simulink model "BuckBosstConverter"  (R2020a)
settings: Solver=FixedStepDiscrete  StartTime=0.0  StopTime=T  FixedStep=Ts  RelTol=1e-3
PreLoadFcn:
  | % Load all configuration
  | config;
values from neighbouring files (symbols this model uses):
  C = 3330e-6    (= 0.00333)    [config.m]
  C_PV = 0.05    [GridConnectedDesignConfiguration.m]    (also in config.m = 0.0001)
  L = 5e-3    (= 0.005)    [config.m]
  LOAD = 7    [config.m]
  R_PV = 10e-3    (= 0.01)    [GridConnectedDesignConfiguration.m]    (also in config.m)
  Rs = 0.1    [config.m]
  temp = 25    [config.m]
  Ts = 5e-6    (= 5e-06)    [GridConnectedDesignConfiguration.m]    (also in config.m = 1e-05)
undefined symbols (not defined in the file or in its folder): Ion, Lithium
libraries: powerlib x13, simulink x2, powerlib_meascontrol x2, electricdrivelib x1, re_lib x1, SignalEditorBlockLib x1
settings Model: Creator=debma  LastModifiedBy=debma

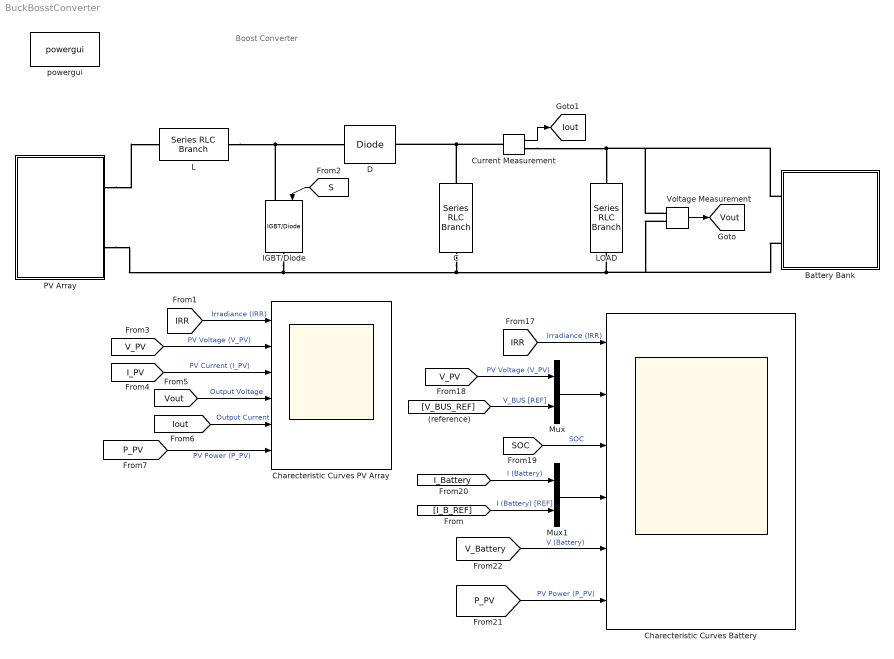
== system BuckBosstConverter ==
  note: Boost Converter
  Battery Bank : Subsystem
  C : powerlib/Elements/Series RLC Branch  LConnTagsString=__new0  RConnTagsString=__new0  BranchType=RC  Resistance=Rs  Inductance=L  SetiL0=off  InitialCurrent=0  Capacitance=C  Setx0=off  InitialVoltage=0  Measurements=None
  Charecteristic Curves Battery : Scope  NumInputPorts=6
  Charecteristic Curves PV Array : Scope  NumInputPorts=6
  Current Measurement : powerlib/Measurements/Current Measurement  PhasorSimulation=off  OutputType=Complex  PSBequivalent=0
  D : powerlib/Power Electronics/Diode  Ron=0.001  Lon=0  Vf=0.8  IC=0  UseSnubber=0  Rs=500  Cs=250e-9  Measurements=off
  IGBT/Diode : powerlib/Power Electronics/IGBT//Diode  Ron=1e-3  Rs=1e5  Cs=inf  Measurements=off
  L : powerlib/Elements/Series RLC Branch  LConnTagsString=__new0  RConnTagsString=__new0  BranchType=RL  Resistance=Rs  Inductance=L  SetiL0=off  InitialCurrent=0  Capacitance=1e-6  Setx0=off  InitialVoltage=0  Measurements=None
  LOAD : powerlib/Elements/Series RLC Branch  LConnTagsString=__new0  RConnTagsString=__new0  BranchType=R  Resistance=LOAD  Inductance=L  SetiL0=off  InitialCurrent=0  Capacitance=1e-6  Setx0=off  InitialVoltage=0  Measurements=None
  Mux : Mux  Inputs=2
  Mux1 : Mux  Inputs=2
  PV Array : Subsystem
  Voltage Measurement : powerlib/Measurements/Voltage Measurement  PhasorSimulation=off  OutputType=Complex  PSBequivalent=0
  powergui : powerlib/powergui  Priority=1  SimulationMode=Discrete  SampleTime=Ts  frequency=60  Iterations=50  frequencyindice=0  Pbase=100e6  ErrMax=1e-4  UnitsV=kV  UnitsW=MW  buscounter=0  FunctionMessages=off  echomessages=off  EnableUseOfTLC=off  CurrentSourceSwitches=off  DisableSnubberDevices=off  DisableRonSwitches=off  DisableVfSwitches=off  DisplayEquations=off  AutomaticDiscreteSolvers=off  SolverType=Tustin/Backward Euler (TBE)  Interpol=off  ExternalGateDelay=off  methode=off  Ts=100  x0status=blocks  SPID=on  SwTol=0  HookPort=off  NonlinearTolerance=1e-4  nMaxIteration=100  ContinueOnMaxIteration=off  RestoreLinks=warning  ResistiveCurrentMeasurement=off  Frange=[0:2:500]  Ylog=off  Xlog=on  ShowGrid=off  save=off  variable=ZData  structure=0  ZoomFFT=off  StartTime=0.0  cycles=1  DisplayStyle=1  fundamental=60  FreqAxis=off  MaxFrequency=1000  frequencyindicesteady=1  RmsSteady=1  display=off
  tag scope: Iout=global, Vout=global
  wires:
  Voltage Measurement/1 -> [Vout]
  Current Measurement/1 -> [Iout]
  [S] -> IGBT/Diode/1
  [V_PV] -> Charecteristic Curves PV Array/2  "PV Voltage (V_PV)"
  [IRR] -> Charecteristic Curves PV Array/1  "Irradiance (IRR)"
  [Vout] -> Charecteristic Curves PV Array/4  "Output Voltage"
  [Iout] -> Charecteristic Curves PV Array/5  "Output Current"
  [I_PV] -> Charecteristic Curves PV Array/3  "PV Current (I_PV)"
  [P_PV] -> Charecteristic Curves PV Array/6  "PV Power (P_PV)"
  Mux/1 -> Charecteristic Curves Battery/2
  [IRR] -> Charecteristic Curves Battery/1  "Irradiance (IRR)"
  [V_BUS_REF] -> Mux/2  "V_BUS [REF]"
  [I_B_REF] -> Mux1/2  "I (Battery) [REF]"
  [SOC] -> Charecteristic Curves Battery/3  "SOC"
  [I_Battery] -> Mux1/1  "I (Battery)"
  [V_Battery] -> Charecteristic Curves Battery/5  "V (Battery)"
  [V_PV] -> Mux/1  "PV Voltage (V_PV)"
  [P_PV] -> Charecteristic Curves Battery/6  "PV Power (P_PV)"
  Mux1/1 -> Charecteristic Curves Battery/4
  connections:
  PV Array/RConn1 -- L/LConn1
  PV Array/RConn2 -- IGBT/Diode/RConn1 -- Voltage Measurement/LConn2 -- Battery Bank/LConn2 -- LOAD/RConn1 -- C/RConn1
  L/RConn1 -- IGBT/Diode/LConn1 -- D/LConn1
  C/LConn1 -- D/RConn1 -- Current Measurement/LConn1
  Current Measurement/RConn1 -- Voltage Measurement/LConn1 -- Battery Bank/LConn1 -- LOAD/LConn1

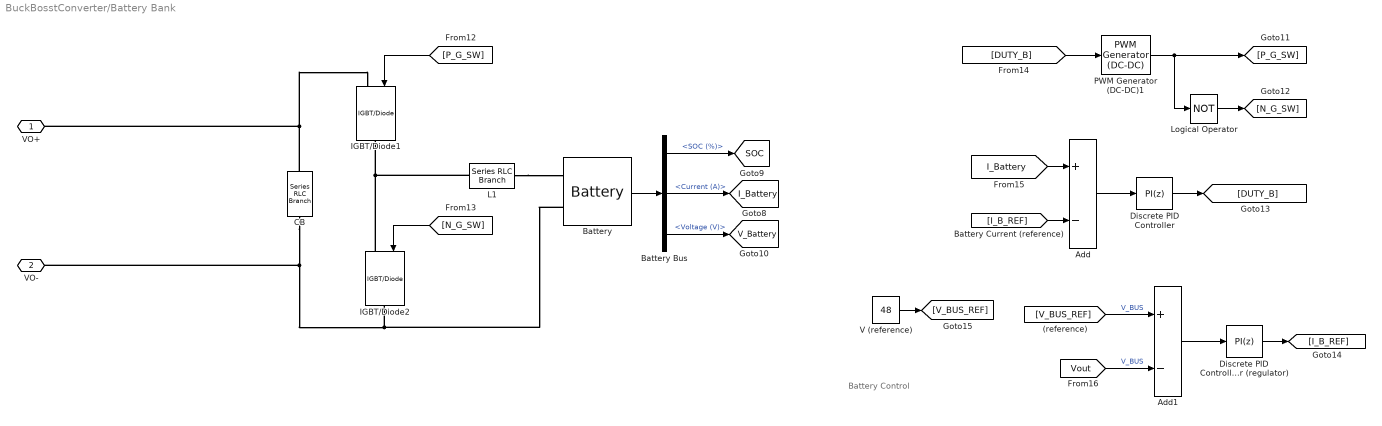
== system BuckBosstConverter/Battery Bank ==
  note: Battery Control
  Add : Sum  Inputs=+-
  Add1 : Sum  Inputs=+-
  Battery : electricdrivelib/Extra Sources/Battery  BatType=Lithium-Ion  ShowTempParam=off  ThermalPreset=no  ShowAgeParam=off  NomV=24  NomQ=50  SOC=45  Batt_Tr=1  PresetModel=on  MaxQ=50  MinV=18  FullV=27.9357  Dis_rate=21.7391  R=0.0048  Normal_OP=45.2174  expZone="[25.9293      2.45652]"  current=[6.5 13 32.5]  Units=Time  Tci=20  NomT=20  T2=-30  MaxQ2=4.8  FullV2=7.1  Normal_OP2=5.655  expZone2="[6.58           1]"  Rca=0.6  ti=2000  Dp=0  Neq0=0  Tsim=1e6  Ta1=25  Qeol=5.4*0.9  Reol=0.013333*1.2  Char_age=[2.3478, 3]  Dis_age=[2.3478, 10]  N1=1500  N2=10500  N3=1000  N4=1400  Ta2=45  N5=950
  Battery Bus : BusSelector  OutputSignals=SOC (%),Current (A),Voltage (V)
  CB : powerlib/Elements/Series RLC Branch  LConnTagsString=__new0  RConnTagsString=__new0  BranchType=RC  Resistance=1e-4  Inductance=1e-3  SetiL0=off  InitialCurrent=0  Capacitance=1000e-6  Setx0=off  InitialVoltage=0  Measurements=None
  Discrete PID Controller : simulink/Continuous/PID Controller  Controller=PI  Form=Parallel  TimeDomain=Discrete-time  UseExternalTs=off  SampleTime=50e-6  IntegratorMethod=Forward Euler  FilterMethod=Forward Euler  ControllerParametersSource=internal  P=0.01  I=10  D=0  UseFilter=on  N=100  TunerSelectOption=Transfer Function Based (PID Tuner App)  InitialConditionSource=internal  InitialConditionForIntegrator=0  InitialConditionForFilter=0  DifferentiatorICPrevScaledInput=0  ExternalReset=none  TrackingMode=off  Kt=1  LimitOutput=on  UpperSaturationLimit=0.95  LowerSaturationLimit=0  LinearizeAsGain=off  AntiWindupMode=none  Kb=1  POutMin=[]  POutMax=[]  IOutMin=[]  IOutMax=[]  DOutMin=[]  DOutMax=[]  NOutMin=[]  NOutMax=[]  SumOutMin=[]  SumOutMax=[]  SaturationOutMin=[]  SaturationOutMax=[]  PParamMin=[]  PParamMax=[]  IParamMin=[]  IParamMax=[]  DParamMin=[]  DParamMax=[]  NParamMin=[]  NParamMax=[]  KbParamMin=[]  KbParamMax=[]  KtParamMin=[]  KtParamMax=[]  KbOutMin=[]  KbOutMax=[]  KtOutMin=[]  KtOutMax=[]  IntegratorOutMin=[]  IntegratorOutMax=[]  FilterOutMin=[]  FilterOutMax=[]  SumI1OutMin=[]  SumI1OutMax=[]  SumI2OutMin=[]  SumI2OutMax=[]  SumI3OutMin=[]  SumI3OutMax=[]  SumI4OutMin=[]  SumI4OutMax=[]  SumDOutMin=[]  SumDOutMax=[]  DifferentiatorOutMin=[]  DifferentiatorOutMax=[]  FilterDiffOutCoefMin=[]  FilterDiffOutCoefMax=[]  ReciprocalOutMin=[]  ReciprocalOutMax=[]  SumDenOutMin=[]  SumDenOutMax=[]  SumNumOutMin=[]  SumNumOutMax=[]  DivideOutMin=[]  DivideOutMax=[]  UdiffTsProdOutMin=[]  UdiffTsProdOutMax=[]  NTsProdOutMin=[]  NTsProdOutMax=[]  UintegralTsProdOutMin=[]  UintegralTsProdOutMax=[]  UngainTsProdOutMin=[]  UngainTsProdOutMax=[]  IntegratorContinuousStateAttributes=''  IntegratorStateMustResolveToSignalObject=off  IntegratorRTWStateStorageClass=Auto  FilterContinuousStateAttributes=''  FilterStateMustResolveToSignalObject=off  FilterRTWStateStorageClass=Auto  ParallelPVariant=InternalParameters  IdealPVariant=Disabled  IVariant=InternalParameters  DVariant=Disabled  IntegratorVariant=Discrete  SatVariant=Enabled  AWVariant=Passthrough  PCopyVariant=Disabled  TRVariant=Disabled  FdbkBlocksVariant=Forward  IdealPFdbkVariant=Disabled  SatFdbkVariant=Disabled  DerivativeFilterVariant=Disabled  NVariant=Disabled  NCopyVariant=Disabled_SignalSpec  FilterICVariant=Disabled  IntegratorICVariant=InternalICs  ExternalResetVariant=Disabled  TRSumVariant=Passthrough  SumFdbkVariant=Disabled  SumVariant=Sum_PI  TsampFilterVariant=InternalTs  TsampNgainVariant=Passthrough  TsampIntegralVariant=Passthrough
  Discrete PID Controller (regulator) : simulink/Continuous/PID Controller  Controller=PI  Form=Parallel  TimeDomain=Discrete-time  UseExternalTs=off  SampleTime=500e-6  IntegratorMethod=Forward Euler  FilterMethod=Forward Euler  ControllerParametersSource=internal  P=0.85  I=10  D=0  UseFilter=on  N=100  TunerSelectOption=Transfer Function Based (PID Tuner App)  InitialConditionSource=internal  InitialConditionForIntegrator=0  InitialConditionForFilter=0  DifferentiatorICPrevScaledInput=0  ExternalReset=none  TrackingMode=off  Kt=1  LimitOutput=on  UpperSaturationLimit=22  LowerSaturationLimit=-22  LinearizeAsGain=off  AntiWindupMode=none  Kb=1  POutMin=[]  POutMax=[]  IOutMin=[]  IOutMax=[]  DOutMin=[]  DOutMax=[]  NOutMin=[]  NOutMax=[]  SumOutMin=[]  SumOutMax=[]  SaturationOutMin=[]  SaturationOutMax=[]  PParamMin=[]  PParamMax=[]  IParamMin=[]  IParamMax=[]  DParamMin=[]  DParamMax=[]  NParamMin=[]  NParamMax=[]  KbParamMin=[]  KbParamMax=[]  KtParamMin=[]  KtParamMax=[]  KbOutMin=[]  KbOutMax=[]  KtOutMin=[]  KtOutMax=[]  IntegratorOutMin=[]  IntegratorOutMax=[]  FilterOutMin=[]  FilterOutMax=[]  SumI1OutMin=[]  SumI1OutMax=[]  SumI2OutMin=[]  SumI2OutMax=[]  SumI3OutMin=[]  SumI3OutMax=[]  SumI4OutMin=[]  SumI4OutMax=[]  SumDOutMin=[]  SumDOutMax=[]  DifferentiatorOutMin=[]  DifferentiatorOutMax=[]  FilterDiffOutCoefMin=[]  FilterDiffOutCoefMax=[]  ReciprocalOutMin=[]  ReciprocalOutMax=[]  SumDenOutMin=[]  SumDenOutMax=[]  SumNumOutMin=[]  SumNumOutMax=[]  DivideOutMin=[]  DivideOutMax=[]  UdiffTsProdOutMin=[]  UdiffTsProdOutMax=[]  NTsProdOutMin=[]  NTsProdOutMax=[]  UintegralTsProdOutMin=[]  UintegralTsProdOutMax=[]  UngainTsProdOutMin=[]  UngainTsProdOutMax=[]  IntegratorContinuousStateAttributes=''  IntegratorStateMustResolveToSignalObject=off  IntegratorRTWStateStorageClass=Auto  FilterContinuousStateAttributes=''  FilterStateMustResolveToSignalObject=off  FilterRTWStateStorageClass=Auto  ParallelPVariant=InternalParameters  IdealPVariant=Disabled  IVariant=InternalParameters  DVariant=Disabled  IntegratorVariant=Discrete  SatVariant=Enabled  AWVariant=Passthrough  PCopyVariant=Disabled  TRVariant=Disabled  FdbkBlocksVariant=Forward  IdealPFdbkVariant=Disabled  SatFdbkVariant=Disabled  DerivativeFilterVariant=Disabled  NVariant=Disabled  NCopyVariant=Disabled_SignalSpec  FilterICVariant=Disabled  IntegratorICVariant=InternalICs  ExternalResetVariant=Disabled  TRSumVariant=Passthrough  SumFdbkVariant=Disabled  SumVariant=Sum_PI  TsampFilterVariant=InternalTs  TsampNgainVariant=Passthrough  TsampIntegralVariant=Passthrough
  IGBT/Diode1 : powerlib/Power Electronics/IGBT//Diode  Ron=1e-3  Rs=1e5  Cs=inf  Measurements=off
  IGBT/Diode2 : powerlib/Power Electronics/IGBT//Diode  Ron=1e-3  Rs=1e5  Cs=inf  Measurements=off
  L1 : powerlib/Elements/Series RLC Branch  LConnTagsString=__new0  RConnTagsString=__new0  BranchType=RL  Resistance=0.1  Inductance=0.5e-3  SetiL0=off  InitialCurrent=0  Capacitance=100e-6  Setx0=off  InitialVoltage=0  Measurements=None
  Logical Operator : Logic  Operator=NOT  AllPortsSameDT=off  OutDataTypeStr=boolean
  PWM Generator (DC-DC)1 : powerlib_meascontrol/Pulse & Signal Generators/PWM Generator (DC-DC)  Fsw=5000  Ts=10e-6
  V (reference) : Constant  Value=48
  VO+ : PMIOPort  Side=Left
  VO- : PMIOPort  Port=2  Side=Left
  tag scope: I_Battery=global, SOC=global, V_Battery=global
  wires:
  Battery Bus/2 -> [I_Battery]  "<Current (A)>"
  Battery/1 -> Battery Bus/1
  Battery Bus/3 -> [V_Battery]  "<Voltage (V)>"
  [N_G_SW] -> IGBT/Diode2/1
  Battery Bus/1 -> [SOC]  "<SOC (%)>"
  [P_G_SW] -> IGBT/Diode1/1
  [I_B_REF] -> Add/2
  [I_Battery] -> Add/1
  [Vout] -> Add1/2  "V_BUS"
  Add/1 -> Discrete PID Controller/1
  [V_BUS_REF] -> Add1/1  "V_BUS"
  V (reference)/1 -> [V_BUS_REF]
  [DUTY_B] -> PWM Generator (DC-DC)1/1
  Logical Operator/1 -> [N_G_SW]
  PWM Generator (DC-DC)1/1 -> Logical Operator/1, [P_G_SW]
  Discrete PID Controller/1 -> [DUTY_B]
  Discrete PID Controller (regulator)/1 -> [I_B_REF]
  Add1/1 -> Discrete PID Controller (regulator)/1
  connections:
  L1/LConn1 -- IGBT/Diode2/LConn1 -- IGBT/Diode1/RConn1
  Battery/LConn2 -- CB/RConn1 -- VO-/RConn1 -- IGBT/Diode2/RConn1
  IGBT/Diode1/LConn1 -- CB/LConn1 -- VO+/RConn1
  L1/RConn1 -- Battery/LConn1

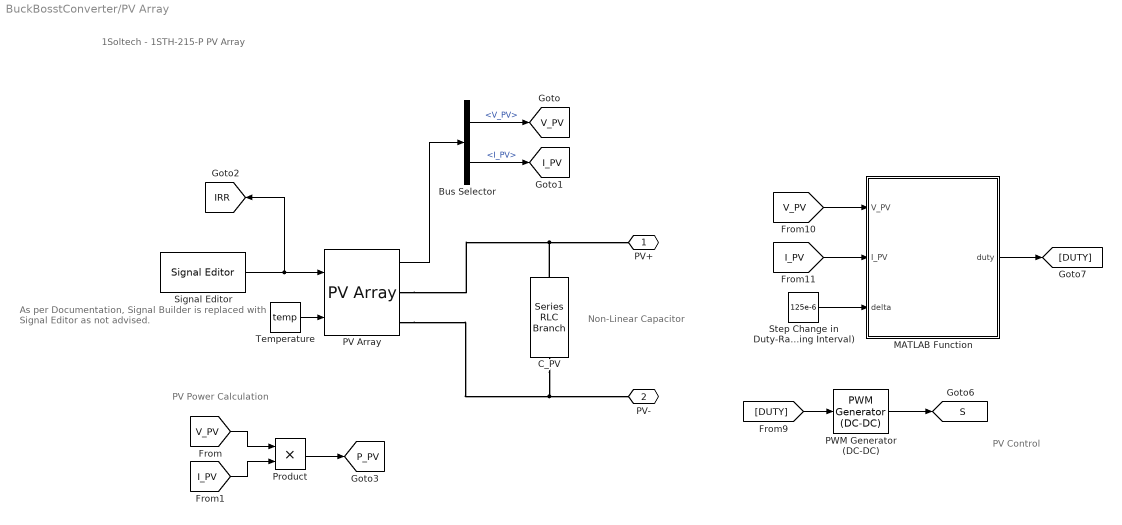
== system BuckBosstConverter/PV Array ==
  note: PV Power Calculation
  note: As per Documentation, Signal Builder is
      | replaced with Signal Editor as not advised.
  note: 1Soltech - 1STH-215-P PV Array
  note: Non-Linear Capacitor
  note: PV Control
  Bus Selector : BusSelector  OutputSignals=V_PV,I_PV
  C_PV : powerlib/Elements/Series RLC Branch  LConnTagsString=__new0  RConnTagsString=__new0  BranchType=RC  Resistance=R_PV  Inductance=1e-3  SetiL0=off  InitialCurrent=0  Capacitance=C_PV  Setx0=off  InitialVoltage=0  Measurements=None
  MATLAB Function : MATLAB Function  TreatAsAtomicUnit=on
  PV Array : re_lib/Solar/PV Array  Npar=5  Nser=1  PlotType=array @ 1000 W/m2 & specified temperatures  S_vec="[ 1000  500  100 ]"  Temp_C_vec="[ 45 25  ]"  ModuleName=1Soltech 1STH-215-P  PlotWhenSelected=off  Pm=213.15  Ncell=60  Voc=36.3  Isc=7.84  Vm=29  Im=7.35  beta_Voc_pc=-0.36099  alpha_Isc_pc=0.102  beta_Voc=-0.13104  alpha_Isc=0.007997  IL=7.8649  I0=2.9259e-10  nI=0.98117  Rsh=313.3991  Rs=0.39383  RobustModel=off  RobustCellTemperature=25  BAL=on  Tc=1e-6  Tfilter=5e-5
  PWM Generator (DC-DC) : powerlib_meascontrol/Pulse & Signal Generators/PWM Generator (DC-DC)  Fsw=5000  Ts=10e-6
  Product : Product
  Signal Editor : SignalEditorBlockLib/Signal Editor  FileName=direct_radiation.mat  ActiveScenario=Scenario  ActiveSignal=radiation  IsBus=off  OutputBusObjectStr=Bus: BusObject  SampleTime=0  ZeroCross=off  OutputAfterFinalValue=Setting to zero  Unit=kW/m^2  PreserveSignalName=on
  Step Change in Duty-Ratio (for Each Sampling Interval) : Constant  Value=125e-6
  Temperature : Constant  Value=temp
  PV+ : PMIOPort  Side=Right
  PV- : PMIOPort  Port=2  Side=Right
  tag scope: IRR=global, I_PV=global, P_PV=global, S=global, V_PV=global
  wires:
  Temperature/1 -> PV Array/2
  Bus Selector/2 -> [I_PV]  "<I_PV>"
  PV Array/1 -> Bus Selector/1
  Bus Selector/1 -> [V_PV]  "<V_PV>"
  Signal Editor/1 -> [IRR], PV Array/1
  [V_PV] -> Product/1
  [I_PV] -> Product/2
  Product/1 -> [P_PV]
  [I_PV] -> MATLAB Function/2(I_PV)
  MATLAB Function/1(duty) -> [DUTY]
  [DUTY] -> PWM Generator (DC-DC)/1
  Step Change in Duty-Ratio (for Each Sampling Interval)/1 -> MATLAB Function/3(delta)
  [V_PV] -> MATLAB Function/1(V_PV)
  PWM Generator (DC-DC)/1 -> [S]
  connections:
  PV Array/RConn1 -- PV+/RConn1 -- C_PV/LConn1
  PV Array/RConn2 -- C_PV/RConn1 -- PV-/RConn1

== matlab function BuckBosstConverter/PV Array/MATLAB Function ==
  data: V_PV input; duty output; I_PV input; delta input
%% MPPT Algorithm, as given by Naki GÜLER in his Video
function duty = MPPT_Algorithm(V_PV, I_PV, delta)
    % First, define the initial Duty Ratio (D)
    D_INIT = 0.05;
    % A min & max D is defined
    D_MIN = 0;
    D_MAX = 0.75;
    
    persistent V_OLD P_OLD D_OLD; % defined, so that these variables,
    % can be accessed everytime, and the old value can be obtained by the
    % difference the old and the new value.
    if isempty(V_OLD)
        V_OLD = 0;
        P_OLD = 0;
        D_OLD = D_INIT;
    end
    
    P = V_PV * I_PV; % Calculated Power
    
    % Calculating delta values, for MPPT Algorithm
    dV = V_PV - V_OLD;
    dP = P - P_OLD;
    
    %% P&O Method of MPPT Tracking Algorithm
    if dP ~= 0 && V_PV > 30
        if dP < 0
            if dV < 0
                duty = D_OLD - delta;
            else
                duty = D_OLD + delta;
            end
        else
            if dV < 0
                duty = D_OLD + delta;
            else
                duty = D_OLD - delta;
            end
        end
    else
        duty = D_OLD;
    end
    
    if duty >= D_MAX
        duty = D_MAX;
    elseif duty < D_MIN
        duty = D_MIN;
    end
    
    %% Setting the OLD Values with the Current Condition Value
    D_OLD = duty;
    V_OLD = V_PV;
    P_OLD = P;
